simulink model "warp_timer"  (Simulink 7.1)
settings: Solver=ode45  StartTime=0.0  StopTime=1000  RelTol=1e-3
undefined symbols (not defined in the file): gcbh, xlBlockLoadCallback, xlGetSimulinkPeriod
libraries: xbsIndex_r4 x450
(part 4 of 5)

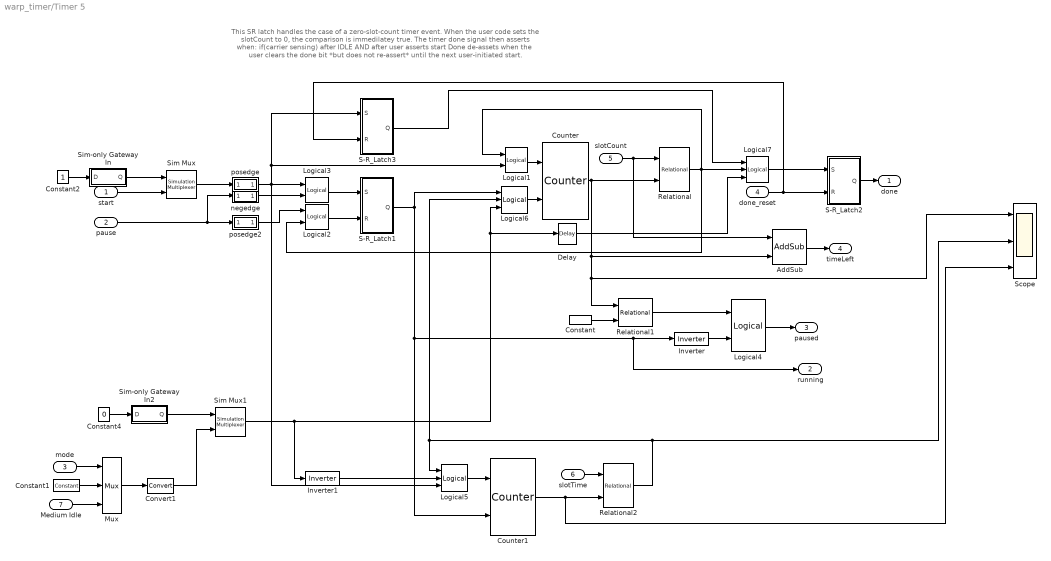
== system warp_timer/Timer 5 ==
  note: This SR latch handles the case of a zero-slot-count
      | timer event. When the user code sets the slotCount to 0,
      | the comparison is immedilatey true. The timer done
      | signal then asserts when:
      | if(carrier sensing) after IDLE AND
      | after user asserts start
      | Done de-assets when the user clears the done bit
      | *but does not re-assert* until the next user-initiated start.
  start : Inport  OutDataType=sfix(16)  OutScaling=2^0
  pause : Inport  Port=2  OutDataType=sfix(16)  OutScaling=2^0
  mode : Inport  Port=3  OutDataType=sfix(16)  OutScaling=2^0
  done_reset : Inport  Port=4  OutDataType=sfix(16)  OutScaling=2^0
  slotCount : Inport  Port=5  OutDataType=sfix(16)  OutScaling=2^0
  slotTime : Inport  Port=6  OutDataType=sfix(16)  OutScaling=2^0
  Medium Idle : Inport  Port=7  OutDataType=sfix(16)  OutScaling=2^0
  AddSub : xbsIndex_r4/AddSub  mode=Subtraction  use_carryin=off  use_carryout=off  en=off  latency=0  precision=User Defined  arith_type=Unsigned  n_bits=32  bin_pt=0  quantization=Truncate  overflow=Wrap  dbl_ovrd=off  use_behavioral_HDL=off  pipelined=off  use_rpm=on  hw_selection=Fabric  block_type=addsub
      settings: xl_area=[16 0 0 32 0 0 0]  block_version=8.2
  Constant : xbsIndex_r4/Constant  arith_type=Unsigned  const=0  n_bits=32  bin_pt=0  explicit_period=off  period=1  equ=P=C  opselect=C  inp2=PCIN>>17  opr=+  inp1=P  carry=CIN  dbl_ovrd=off  block_type=constant
      settings: block_version=10.1.2
  Constant1 : xbsIndex_r4/Constant  arith_type=Unsigned  const=1  n_bits=1  bin_pt=0  explicit_period=off  period=1  equ=P=C  opselect=C  inp2=PCIN>>17  opr=+  inp1=P  carry=CIN  dbl_ovrd=off  block_type=constant
      settings: block_version=8.2
  Constant2 : Constant  OutDataType=sfix(16)  OutScaling=2^0
  Constant4 : Constant  Value=0  OutDataType=sfix(16)  OutScaling=2^0
  Convert1 : xbsIndex_r4/Convert  arith_type=Boolean  n_bits=16  bin_pt=14  quantization=Truncate  overflow=Wrap  latency=0  dbl_ovrd=off  pipeline=off  block_type=convert
      settings: xl_area=[0 0 0 0 0 0 0]  block_version=8.2
  Counter : xbsIndex_r4/Counter  cnt_type=Free Running  cnt_to=Inf  operation=Up  start_count=0  cnt_by_val=1  arith_type=Unsigned  n_bits=32  bin_pt=0  load_pin=off  rst=on  en=on  explicit_period=on  period=1  dbl_ovrd=off  use_behavioral_HDL=off  use_rpm=off  implementation=Fabric  block_type=counter
      settings: xl_area=[17 32 0 32 0 0 0]  block_version=8.2
  Counter1 : xbsIndex_r4/Counter  cnt_type=Free Running  cnt_to=Inf  operation=Up  start_count=0  cnt_by_val=1  arith_type=Unsigned  n_bits=16  bin_pt=0  load_pin=off  rst=on  en=on  explicit_period=on  period=1  dbl_ovrd=off  use_behavioral_HDL=off  use_rpm=off  implementation=Fabric  block_type=counter
      settings: xl_area=[17 32 0 32 0 0 0]  block_version=8.2
  Delay : xbsIndex_r4/Delay  en=off  latency=1  dbl_ovrd=off  reg_retiming=off  block_type=delay
  Inverter : xbsIndex_r4/Inverter  en=off  latency=0  dbl_ovrd=off  block_type=inv
      settings: xl_area=[0 0 0 0 0 0 0]  block_version=10.1.2
  Inverter1 : xbsIndex_r4/Inverter  en=off  latency=0  dbl_ovrd=off  block_type=inv
      settings: xl_area=[0 0 0 0 0 0 0]  block_version=10.1.2
  Logical1 : xbsIndex_r4/Logical  logical_function=OR  inputs=2  en=off  latency=0  precision=Full  arith_type=Unsigned  n_bits=16  bin_pt=0  align_bp=on  dbl_ovrd=off  block_type=logical
      settings: xl_area=[1 0 0 1 0 0 0]  block_version=9.1.01
  Logical2 : xbsIndex_r4/Logical  logical_function=OR  inputs=2  en=off  latency=0  precision=Full  arith_type=Unsigned  n_bits=16  bin_pt=0  align_bp=on  dbl_ovrd=off  block_type=logical
      settings: xl_area=[1 0 0 1 0 0 0]  block_version=9.1.01
  Logical3 : xbsIndex_r4/Logical  logical_function=OR  inputs=2  en=off  latency=0  precision=Full  arith_type=Unsigned  n_bits=16  bin_pt=0  align_bp=on  dbl_ovrd=off  block_type=logical
      settings: xl_area=[1 0 0 1 0 0 0]  block_version=9.1.01
  Logical4 : xbsIndex_r4/Logical  logical_function=AND  inputs=2  en=off  latency=0  precision=Full  arith_type=Unsigned  n_bits=16  bin_pt=0  align_bp=on  dbl_ovrd=off  block_type=logical
      settings: xl_area=[1 0 0 1 0 0 0]  block_version=10.1.2
  Logical5 : xbsIndex_r4/Logical  logical_function=OR  inputs=3  en=off  latency=0  precision=Full  arith_type=Unsigned  n_bits=16  bin_pt=0  align_bp=on  dbl_ovrd=off  block_type=logical
      settings: xl_area=[1 0 0 1 0 0 0]  block_version=8.2
  Logical6 : xbsIndex_r4/Logical  logical_function=AND  inputs=3  en=off  latency=0  precision=Full  arith_type=Unsigned  n_bits=16  bin_pt=0  align_bp=on  dbl_ovrd=off  block_type=logical
      settings: xl_area=[1 0 0 1 0 0 0]  block_version=8.2
  Logical7 : xbsIndex_r4/Logical  logical_function=AND  inputs=3  en=off  latency=0  precision=Full  arith_type=Unsigned  n_bits=16  bin_pt=0  align_bp=on  dbl_ovrd=off  block_type=logical
      settings: xl_area=[1 0 0 1 0 0 0]  block_version=9.1.01
  Mux : xbsIndex_r4/Mux  inputs=2  en=off  latency=0  precision=Full  arith_type=Unsigned  n_bits=16  bin_pt=14  quantization=Truncate  overflow=Wrap  dbl_ovrd=off  block_type=mux
      settings: xl_area=[1 0 0 1 0 0 0]  block_version=8.2
  Relational : xbsIndex_r4/Relational  mode=a<=b  en=off  latency=0  dbl_ovrd=off  block_type=relational
      settings: xl_area=[8 0 0 16 0 0 0]  block_version=8.2
  Relational1 : xbsIndex_r4/Relational  mode=a>b  en=off  latency=0  dbl_ovrd=off  block_type=relational
      settings: xl_area=[16 1 0 32 0 0 0]  block_version=10.1.2
  Relational2 : xbsIndex_r4/Relational  mode=a<=b  en=off  latency=0  dbl_ovrd=off  block_type=relational
      settings: xl_area=[8 0 0 16 0 0 0]  block_version=8.2
  S-R_Latch1 : Subsystem
  S-R_Latch2 : Subsystem
  S-R_Latch3 : Subsystem
  Scope : Scope  NumInputPorts=3
      settings: YMin=-5~-5~-5  YMax=5~5~5
  Sim Mux : xbsIndex_r4/Simulation Multiplexer  sim_sel=1  hw_sel=2  block_type=simmux
      settings: infoedit="Distinguish input subsystems as \"simulation only\" and \"generation only\".  The input specified For Simulation will be used during Simulink simulation.  The input specified For Generation will be used during code generation.  This block will typically be used on the output of a HW Co-Simulation, Black Box, or ModelSim subsystem.<P><P>Hardware Notes: This block costs nothing."  block_version=10.1.3
  Sim Mux1 : xbsIndex_r4/Simulation Multiplexer  sim_sel=1  hw_sel=2  block_type=simmux
      settings: infoedit="Distinguish input subsystems as \"simulation only\" and \"generation only\".  The input specified For Simulation will be used during Simulink simulation.  The input specified For Generation will be used during code generation.  This block will typically be used on the output of a HW Co-Simulation, Black Box, or ModelSim subsystem.<P><P>Hardware Notes: This block costs nothing."  block_version=10.1.3
  Sim-only Gateway In : Subsystem
  Sim-only Gateway In2 : Subsystem
  negedge : Subsystem
  posedge : Subsystem
  posedge2 : Subsystem
  done : Outport  OutDataType=sfix(16)  OutScaling=2^0
  running : Outport  Port=2  OutDataType=sfix(16)  OutScaling=2^0
  paused : Outport  Port=3  OutDataType=sfix(16)  OutScaling=2^0
  timeLeft : Outport  Port=4  OutDataType=sfix(16)  OutScaling=2^0
  wires:
  Delay/1 -> Logical7/3
  S-R_Latch3/1(Q) -> Logical7/1
  Logical7/1 -> S-R_Latch2/1(S)
  Sim-only Gateway In2/1(Q) -> Sim Mux1/1
  Constant4/1 -> Sim-only Gateway In2/1(D)
  Logical2/1 -> S-R_Latch1/2(R)
  posedge2/1(Out) -> Logical2/1
  Constant2/1 -> Sim-only Gateway In/1(D)
  Sim Mux1/1 -> Delay/1, Logical6/3, Inverter1/1
  Convert1/1 -> Sim Mux1/2
  Logical6/1 -> Counter/2
  Inverter1/1 -> Logical5/2
  Relational2/1 -> Scope/2, Logical6/2, Logical5/1
  Logical5/1 -> Counter1/1
  Counter1/1 -> Scope/3, Relational2/2
  slotTime/1 -> Relational2/1
  Sim-only Gateway In/1(Q) -> Sim Mux/1
  pause/1 -> negedge/1(In), posedge2/1(In)
  negedge/1(Out) -> Logical3/2
  Logical3/1 -> S-R_Latch1/1(S)
  posedge/1(Out) -> S-R_Latch3/1(S), Logical1/2, Logical5/3, Logical3/1
  done_reset/1 -> S-R_Latch3/2(R), S-R_Latch2/2(R)
  Relational/1 -> Logical7/2, Logical1/1, Logical2/2
  S-R_Latch2/1(Q) -> done/1
  Logical1/1 -> Counter/1
  Counter/1 -> Scope/1, Relational1/1, AddSub/2, Relational/2
  slotCount/1 -> Relational/1, AddSub/1
  S-R_Latch1/1(Q) -> Logical6/1, running/1, Inverter/1, Counter1/2
  Inverter/1 -> Logical4/2
  Relational1/1 -> Logical4/1
  Constant/1 -> Relational1/2
  AddSub/1 -> timeLeft/1
  Sim Mux/1 -> posedge/1(In)
  start/1 -> Sim Mux/2
  Logical4/1 -> paused/1
  Mux/1 -> Convert1/1
  Medium Idle/1 -> Mux/3
  Constant1/1 -> Mux/2
  mode/1 -> Mux/1

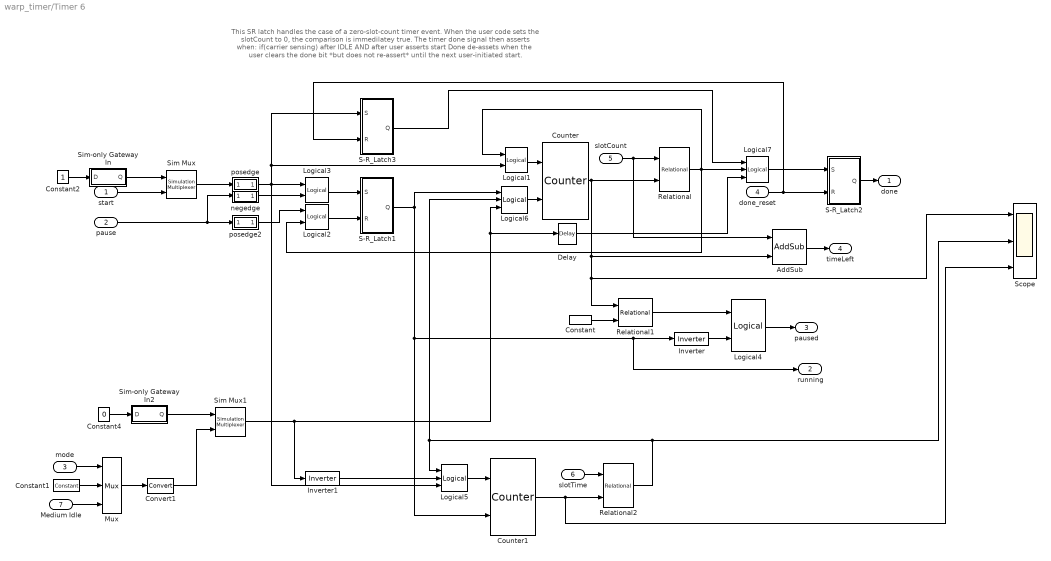
== system warp_timer/Timer 6 ==
  note: This SR latch handles the case of a zero-slot-count
      | timer event. When the user code sets the slotCount to 0,
      | the comparison is immedilatey true. The timer done
      | signal then asserts when:
      | if(carrier sensing) after IDLE AND
      | after user asserts start
      | Done de-assets when the user clears the done bit
      | *but does not re-assert* until the next user-initiated start.
  start : Inport  OutDataType=sfix(16)  OutScaling=2^0
  pause : Inport  Port=2  OutDataType=sfix(16)  OutScaling=2^0
  mode : Inport  Port=3  OutDataType=sfix(16)  OutScaling=2^0
  done_reset : Inport  Port=4  OutDataType=sfix(16)  OutScaling=2^0
  slotCount : Inport  Port=5  OutDataType=sfix(16)  OutScaling=2^0
  slotTime : Inport  Port=6  OutDataType=sfix(16)  OutScaling=2^0
  Medium Idle : Inport  Port=7  OutDataType=sfix(16)  OutScaling=2^0
  AddSub : xbsIndex_r4/AddSub  mode=Subtraction  use_carryin=off  use_carryout=off  en=off  latency=0  precision=User Defined  arith_type=Unsigned  n_bits=32  bin_pt=0  quantization=Truncate  overflow=Wrap  dbl_ovrd=off  use_behavioral_HDL=off  pipelined=off  use_rpm=on  hw_selection=Fabric  block_type=addsub
      settings: xl_area=[16 0 0 32 0 0 0]  block_version=8.2
  Constant : xbsIndex_r4/Constant  arith_type=Unsigned  const=0  n_bits=32  bin_pt=0  explicit_period=off  period=1  equ=P=C  opselect=C  inp2=PCIN>>17  opr=+  inp1=P  carry=CIN  dbl_ovrd=off  block_type=constant
      settings: block_version=10.1.2
  Constant1 : xbsIndex_r4/Constant  arith_type=Unsigned  const=1  n_bits=1  bin_pt=0  explicit_period=off  period=1  equ=P=C  opselect=C  inp2=PCIN>>17  opr=+  inp1=P  carry=CIN  dbl_ovrd=off  block_type=constant
      settings: block_version=8.2
  Constant2 : Constant  OutDataType=sfix(16)  OutScaling=2^0
  Constant4 : Constant  Value=0  OutDataType=sfix(16)  OutScaling=2^0
  Convert1 : xbsIndex_r4/Convert  arith_type=Boolean  n_bits=16  bin_pt=14  quantization=Truncate  overflow=Wrap  latency=0  dbl_ovrd=off  pipeline=off  block_type=convert
      settings: xl_area=[0 0 0 0 0 0 0]  block_version=8.2
  Counter : xbsIndex_r4/Counter  cnt_type=Free Running  cnt_to=Inf  operation=Up  start_count=0  cnt_by_val=1  arith_type=Unsigned  n_bits=32  bin_pt=0  load_pin=off  rst=on  en=on  explicit_period=on  period=1  dbl_ovrd=off  use_behavioral_HDL=off  use_rpm=off  implementation=Fabric  block_type=counter
      settings: xl_area=[17 32 0 32 0 0 0]  block_version=8.2
  Counter1 : xbsIndex_r4/Counter  cnt_type=Free Running  cnt_to=Inf  operation=Up  start_count=0  cnt_by_val=1  arith_type=Unsigned  n_bits=16  bin_pt=0  load_pin=off  rst=on  en=on  explicit_period=on  period=1  dbl_ovrd=off  use_behavioral_HDL=off  use_rpm=off  implementation=Fabric  block_type=counter
      settings: xl_area=[17 32 0 32 0 0 0]  block_version=8.2
  Delay : xbsIndex_r4/Delay  en=off  latency=1  dbl_ovrd=off  reg_retiming=off  block_type=delay
  Inverter : xbsIndex_r4/Inverter  en=off  latency=0  dbl_ovrd=off  block_type=inv
      settings: xl_area=[0 0 0 0 0 0 0]  block_version=10.1.2
  Inverter1 : xbsIndex_r4/Inverter  en=off  latency=0  dbl_ovrd=off  block_type=inv
      settings: xl_area=[0 0 0 0 0 0 0]  block_version=10.1.2
  Logical1 : xbsIndex_r4/Logical  logical_function=OR  inputs=2  en=off  latency=0  precision=Full  arith_type=Unsigned  n_bits=16  bin_pt=0  align_bp=on  dbl_ovrd=off  block_type=logical
      settings: xl_area=[1 0 0 1 0 0 0]  block_version=9.1.01
  Logical2 : xbsIndex_r4/Logical  logical_function=OR  inputs=2  en=off  latency=0  precision=Full  arith_type=Unsigned  n_bits=16  bin_pt=0  align_bp=on  dbl_ovrd=off  block_type=logical
      settings: xl_area=[1 0 0 1 0 0 0]  block_version=9.1.01
  Logical3 : xbsIndex_r4/Logical  logical_function=OR  inputs=2  en=off  latency=0  precision=Full  arith_type=Unsigned  n_bits=16  bin_pt=0  align_bp=on  dbl_ovrd=off  block_type=logical
      settings: xl_area=[1 0 0 1 0 0 0]  block_version=9.1.01
  Logical4 : xbsIndex_r4/Logical  logical_function=AND  inputs=2  en=off  latency=0  precision=Full  arith_type=Unsigned  n_bits=16  bin_pt=0  align_bp=on  dbl_ovrd=off  block_type=logical
      settings: xl_area=[1 0 0 1 0 0 0]  block_version=10.1.2
  Logical5 : xbsIndex_r4/Logical  logical_function=OR  inputs=3  en=off  latency=0  precision=Full  arith_type=Unsigned  n_bits=16  bin_pt=0  align_bp=on  dbl_ovrd=off  block_type=logical
      settings: xl_area=[1 0 0 1 0 0 0]  block_version=8.2
  Logical6 : xbsIndex_r4/Logical  logical_function=AND  inputs=3  en=off  latency=0  precision=Full  arith_type=Unsigned  n_bits=16  bin_pt=0  align_bp=on  dbl_ovrd=off  block_type=logical
      settings: xl_area=[1 0 0 1 0 0 0]  block_version=8.2
  Logical7 : xbsIndex_r4/Logical  logical_function=AND  inputs=3  en=off  latency=0  precision=Full  arith_type=Unsigned  n_bits=16  bin_pt=0  align_bp=on  dbl_ovrd=off  block_type=logical
      settings: xl_area=[1 0 0 1 0 0 0]  block_version=9.1.01
  Mux : xbsIndex_r4/Mux  inputs=2  en=off  latency=0  precision=Full  arith_type=Unsigned  n_bits=16  bin_pt=14  quantization=Truncate  overflow=Wrap  dbl_ovrd=off  block_type=mux
      settings: xl_area=[1 0 0 1 0 0 0]  block_version=8.2
  Relational : xbsIndex_r4/Relational  mode=a<=b  en=off  latency=0  dbl_ovrd=off  block_type=relational
      settings: xl_area=[8 0 0 16 0 0 0]  block_version=8.2
  Relational1 : xbsIndex_r4/Relational  mode=a>b  en=off  latency=0  dbl_ovrd=off  block_type=relational
      settings: xl_area=[16 1 0 32 0 0 0]  block_version=10.1.2
  Relational2 : xbsIndex_r4/Relational  mode=a<=b  en=off  latency=0  dbl_ovrd=off  block_type=relational
      settings: xl_area=[8 0 0 16 0 0 0]  block_version=8.2
  S-R_Latch1 : Subsystem
  S-R_Latch2 : Subsystem
  S-R_Latch3 : Subsystem
  Scope : Scope  NumInputPorts=3
      settings: YMin=-5~-5~-5  YMax=5~5~5
  Sim Mux : xbsIndex_r4/Simulation Multiplexer  sim_sel=1  hw_sel=2  block_type=simmux
      settings: infoedit="Distinguish input subsystems as \"simulation only\" and \"generation only\".  The input specified For Simulation will be used during Simulink simulation.  The input specified For Generation will be used during code generation.  This block will typically be used on the output of a HW Co-Simulation, Black Box, or ModelSim subsystem.<P><P>Hardware Notes: This block costs nothing."  block_version=10.1.3
  Sim Mux1 : xbsIndex_r4/Simulation Multiplexer  sim_sel=1  hw_sel=2  block_type=simmux
      settings: infoedit="Distinguish input subsystems as \"simulation only\" and \"generation only\".  The input specified For Simulation will be used during Simulink simulation.  The input specified For Generation will be used during code generation.  This block will typically be used on the output of a HW Co-Simulation, Black Box, or ModelSim subsystem.<P><P>Hardware Notes: This block costs nothing."  block_version=10.1.3
  Sim-only Gateway In : Subsystem
  Sim-only Gateway In2 : Subsystem
  negedge : Subsystem
  posedge : Subsystem
  posedge2 : Subsystem
  done : Outport  OutDataType=sfix(16)  OutScaling=2^0
  running : Outport  Port=2  OutDataType=sfix(16)  OutScaling=2^0
  paused : Outport  Port=3  OutDataType=sfix(16)  OutScaling=2^0
  timeLeft : Outport  Port=4  OutDataType=sfix(16)  OutScaling=2^0
  wires:
  mode/1 -> Mux/1
  Constant1/1 -> Mux/2
  Medium Idle/1 -> Mux/3
  Mux/1 -> Convert1/1
  Logical4/1 -> paused/1
  start/1 -> Sim Mux/2
  Sim Mux/1 -> posedge/1(In)
  AddSub/1 -> timeLeft/1
  Constant/1 -> Relational1/2
  Relational1/1 -> Logical4/1
  Inverter/1 -> Logical4/2
  S-R_Latch1/1(Q) -> Counter1/2, Inverter/1, running/1, Logical6/1
  slotCount/1 -> AddSub/1, Relational/1
  Counter/1 -> Relational/2, AddSub/2, Relational1/1, Scope/1
  Logical1/1 -> Counter/1
  S-R_Latch2/1(Q) -> done/1
  Relational/1 -> Logical2/2, Logical1/1, Logical7/2
  done_reset/1 -> S-R_Latch2/2(R), S-R_Latch3/2(R)
  posedge/1(Out) -> Logical3/1, Logical5/3, Logical1/2, S-R_Latch3/1(S)
  Logical3/1 -> S-R_Latch1/1(S)
  negedge/1(Out) -> Logical3/2
  pause/1 -> posedge2/1(In), negedge/1(In)
  Sim-only Gateway In/1(Q) -> Sim Mux/1
  slotTime/1 -> Relational2/1
  Counter1/1 -> Relational2/2, Scope/3
  Logical5/1 -> Counter1/1
  Relational2/1 -> Logical5/1, Logical6/2, Scope/2
  Inverter1/1 -> Logical5/2
  Logical6/1 -> Counter/2
  Convert1/1 -> Sim Mux1/2
  Sim Mux1/1 -> Inverter1/1, Logical6/3, Delay/1
  Constant2/1 -> Sim-only Gateway In/1(D)
  posedge2/1(Out) -> Logical2/1
  Logical2/1 -> S-R_Latch1/2(R)
  Constant4/1 -> Sim-only Gateway In2/1(D)
  Sim-only Gateway In2/1(Q) -> Sim Mux1/1
  Logical7/1 -> S-R_Latch2/1(S)
  S-R_Latch3/1(Q) -> Logical7/1
  Delay/1 -> Logical7/3

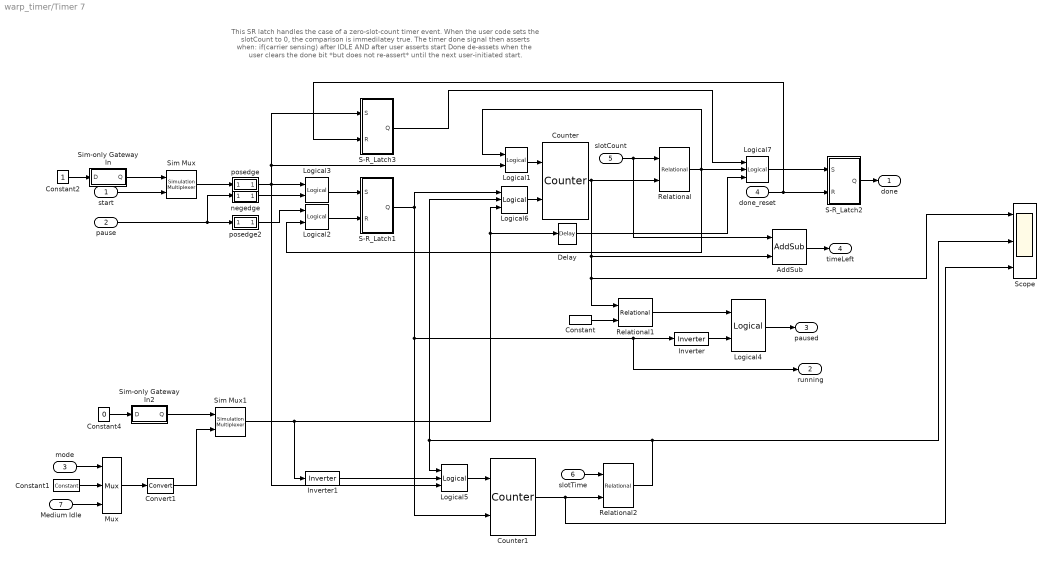
== system warp_timer/Timer 7 ==
  note: This SR latch handles the case of a zero-slot-count
      | timer event. When the user code sets the slotCount to 0,
      | the comparison is immedilatey true. The timer done
      | signal then asserts when:
      | if(carrier sensing) after IDLE AND
      | after user asserts start
      | Done de-assets when the user clears the done bit
      | *but does not re-assert* until the next user-initiated start.
  start : Inport  OutDataType=sfix(16)  OutScaling=2^0
  pause : Inport  Port=2  OutDataType=sfix(16)  OutScaling=2^0
  mode : Inport  Port=3  OutDataType=sfix(16)  OutScaling=2^0
  done_reset : Inport  Port=4  OutDataType=sfix(16)  OutScaling=2^0
  slotCount : Inport  Port=5  OutDataType=sfix(16)  OutScaling=2^0
  slotTime : Inport  Port=6  OutDataType=sfix(16)  OutScaling=2^0
  Medium Idle : Inport  Port=7  OutDataType=sfix(16)  OutScaling=2^0
  AddSub : xbsIndex_r4/AddSub  mode=Subtraction  use_carryin=off  use_carryout=off  en=off  latency=0  precision=User Defined  arith_type=Unsigned  n_bits=32  bin_pt=0  quantization=Truncate  overflow=Wrap  dbl_ovrd=off  use_behavioral_HDL=off  pipelined=off  use_rpm=on  hw_selection=Fabric  block_type=addsub
      settings: xl_area=[16 0 0 32 0 0 0]  block_version=8.2
  Constant : xbsIndex_r4/Constant  arith_type=Unsigned  const=0  n_bits=32  bin_pt=0  explicit_period=off  period=1  equ=P=C  opselect=C  inp2=PCIN>>17  opr=+  inp1=P  carry=CIN  dbl_ovrd=off  block_type=constant
      settings: block_version=10.1.2
  Constant1 : xbsIndex_r4/Constant  arith_type=Unsigned  const=1  n_bits=1  bin_pt=0  explicit_period=off  period=1  equ=P=C  opselect=C  inp2=PCIN>>17  opr=+  inp1=P  carry=CIN  dbl_ovrd=off  block_type=constant
      settings: block_version=8.2
  Constant2 : Constant  OutDataType=sfix(16)  OutScaling=2^0
  Constant4 : Constant  Value=0  OutDataType=sfix(16)  OutScaling=2^0
  Convert1 : xbsIndex_r4/Convert  arith_type=Boolean  n_bits=16  bin_pt=14  quantization=Truncate  overflow=Wrap  latency=0  dbl_ovrd=off  pipeline=off  block_type=convert
      settings: xl_area=[0 0 0 0 0 0 0]  block_version=8.2
  Counter : xbsIndex_r4/Counter  cnt_type=Free Running  cnt_to=Inf  operation=Up  start_count=0  cnt_by_val=1  arith_type=Unsigned  n_bits=32  bin_pt=0  load_pin=off  rst=on  en=on  explicit_period=on  period=1  dbl_ovrd=off  use_behavioral_HDL=off  use_rpm=off  implementation=Fabric  block_type=counter
      settings: xl_area=[17 32 0 32 0 0 0]  block_version=8.2
  Counter1 : xbsIndex_r4/Counter  cnt_type=Free Running  cnt_to=Inf  operation=Up  start_count=0  cnt_by_val=1  arith_type=Unsigned  n_bits=16  bin_pt=0  load_pin=off  rst=on  en=on  explicit_period=on  period=1  dbl_ovrd=off  use_behavioral_HDL=off  use_rpm=off  implementation=Fabric  block_type=counter
      settings: xl_area=[17 32 0 32 0 0 0]  block_version=8.2
  Delay : xbsIndex_r4/Delay  en=off  latency=1  dbl_ovrd=off  reg_retiming=off  block_type=delay
  Inverter : xbsIndex_r4/Inverter  en=off  latency=0  dbl_ovrd=off  block_type=inv
      settings: xl_area=[0 0 0 0 0 0 0]  block_version=10.1.2
  Inverter1 : xbsIndex_r4/Inverter  en=off  latency=0  dbl_ovrd=off  block_type=inv
      settings: xl_area=[0 0 0 0 0 0 0]  block_version=10.1.2
  Logical1 : xbsIndex_r4/Logical  logical_function=OR  inputs=2  en=off  latency=0  precision=Full  arith_type=Unsigned  n_bits=16  bin_pt=0  align_bp=on  dbl_ovrd=off  block_type=logical
      settings: xl_area=[1 0 0 1 0 0 0]  block_version=9.1.01
  Logical2 : xbsIndex_r4/Logical  logical_function=OR  inputs=2  en=off  latency=0  precision=Full  arith_type=Unsigned  n_bits=16  bin_pt=0  align_bp=on  dbl_ovrd=off  block_type=logical
      settings: xl_area=[1 0 0 1 0 0 0]  block_version=9.1.01
  Logical3 : xbsIndex_r4/Logical  logical_function=OR  inputs=2  en=off  latency=0  precision=Full  arith_type=Unsigned  n_bits=16  bin_pt=0  align_bp=on  dbl_ovrd=off  block_type=logical
      settings: xl_area=[1 0 0 1 0 0 0]  block_version=9.1.01
  Logical4 : xbsIndex_r4/Logical  logical_function=AND  inputs=2  en=off  latency=0  precision=Full  arith_type=Unsigned  n_bits=16  bin_pt=0  align_bp=on  dbl_ovrd=off  block_type=logical
      settings: xl_area=[1 0 0 1 0 0 0]  block_version=10.1.2
  Logical5 : xbsIndex_r4/Logical  logical_function=OR  inputs=3  en=off  latency=0  precision=Full  arith_type=Unsigned  n_bits=16  bin_pt=0  align_bp=on  dbl_ovrd=off  block_type=logical
      settings: xl_area=[1 0 0 1 0 0 0]  block_version=8.2
  Logical6 : xbsIndex_r4/Logical  logical_function=AND  inputs=3  en=off  latency=0  precision=Full  arith_type=Unsigned  n_bits=16  bin_pt=0  align_bp=on  dbl_ovrd=off  block_type=logical
      settings: xl_area=[1 0 0 1 0 0 0]  block_version=8.2
  Logical7 : xbsIndex_r4/Logical  logical_function=AND  inputs=3  en=off  latency=0  precision=Full  arith_type=Unsigned  n_bits=16  bin_pt=0  align_bp=on  dbl_ovrd=off  block_type=logical
      settings: xl_area=[1 0 0 1 0 0 0]  block_version=9.1.01
  Mux : xbsIndex_r4/Mux  inputs=2  en=off  latency=0  precision=Full  arith_type=Unsigned  n_bits=16  bin_pt=14  quantization=Truncate  overflow=Wrap  dbl_ovrd=off  block_type=mux
      settings: xl_area=[1 0 0 1 0 0 0]  block_version=8.2
  Relational : xbsIndex_r4/Relational  mode=a<=b  en=off  latency=0  dbl_ovrd=off  block_type=relational
      settings: xl_area=[8 0 0 16 0 0 0]  block_version=8.2
  Relational1 : xbsIndex_r4/Relational  mode=a>b  en=off  latency=0  dbl_ovrd=off  block_type=relational
      settings: xl_area=[16 1 0 32 0 0 0]  block_version=10.1.2
  Relational2 : xbsIndex_r4/Relational  mode=a<=b  en=off  latency=0  dbl_ovrd=off  block_type=relational
      settings: xl_area=[8 0 0 16 0 0 0]  block_version=8.2
  S-R_Latch1 : Subsystem
  S-R_Latch2 : Subsystem
  S-R_Latch3 : Subsystem
  Scope : Scope  NumInputPorts=3
      settings: YMin=-5~-5~-5  YMax=5~5~5
  Sim Mux : xbsIndex_r4/Simulation Multiplexer  sim_sel=1  hw_sel=2  block_type=simmux
      settings: infoedit="Distinguish input subsystems as \"simulation only\" and \"generation only\".  The input specified For Simulation will be used during Simulink simulation.  The input specified For Generation will be used during code generation.  This block will typically be used on the output of a HW Co-Simulation, Black Box, or ModelSim subsystem.<P><P>Hardware Notes: This block costs nothing."  block_version=10.1.3
  Sim Mux1 : xbsIndex_r4/Simulation Multiplexer  sim_sel=1  hw_sel=2  block_type=simmux
      settings: infoedit="Distinguish input subsystems as \"simulation only\" and \"generation only\".  The input specified For Simulation will be used during Simulink simulation.  The input specified For Generation will be used during code generation.  This block will typically be used on the output of a HW Co-Simulation, Black Box, or ModelSim subsystem.<P><P>Hardware Notes: This block costs nothing."  block_version=10.1.3
  Sim-only Gateway In : Subsystem
  Sim-only Gateway In2 : Subsystem
  negedge : Subsystem
  posedge : Subsystem
  posedge2 : Subsystem
  done : Outport  OutDataType=sfix(16)  OutScaling=2^0
  running : Outport  Port=2  OutDataType=sfix(16)  OutScaling=2^0
  paused : Outport  Port=3  OutDataType=sfix(16)  OutScaling=2^0
  timeLeft : Outport  Port=4  OutDataType=sfix(16)  OutScaling=2^0
  wires:
  Delay/1 -> Logical7/3
  S-R_Latch3/1(Q) -> Logical7/1
  Logical7/1 -> S-R_Latch2/1(S)
  Sim-only Gateway In2/1(Q) -> Sim Mux1/1
  Constant4/1 -> Sim-only Gateway In2/1(D)
  Logical2/1 -> S-R_Latch1/2(R)
  posedge2/1(Out) -> Logical2/1
  Constant2/1 -> Sim-only Gateway In/1(D)
  Sim Mux1/1 -> Delay/1, Logical6/3, Inverter1/1
  Convert1/1 -> Sim Mux1/2
  Logical6/1 -> Counter/2
  Inverter1/1 -> Logical5/2
  Relational2/1 -> Scope/2, Logical6/2, Logical5/1
  Logical5/1 -> Counter1/1
  Counter1/1 -> Scope/3, Relational2/2
  slotTime/1 -> Relational2/1
  Sim-only Gateway In/1(Q) -> Sim Mux/1
  pause/1 -> negedge/1(In), posedge2/1(In)
  negedge/1(Out) -> Logical3/2
  Logical3/1 -> S-R_Latch1/1(S)
  posedge/1(Out) -> S-R_Latch3/1(S), Logical1/2, Logical5/3, Logical3/1
  done_reset/1 -> S-R_Latch3/2(R), S-R_Latch2/2(R)
  Relational/1 -> Logical7/2, Logical1/1, Logical2/2
  S-R_Latch2/1(Q) -> done/1
  Logical1/1 -> Counter/1
  Counter/1 -> Scope/1, Relational1/1, AddSub/2, Relational/2
  slotCount/1 -> Relational/1, AddSub/1
  S-R_Latch1/1(Q) -> Logical6/1, running/1, Inverter/1, Counter1/2
  Inverter/1 -> Logical4/2
  Relational1/1 -> Logical4/1
  Constant/1 -> Relational1/2
  AddSub/1 -> timeLeft/1
  Sim Mux/1 -> posedge/1(In)
  start/1 -> Sim Mux/2
  Logical4/1 -> paused/1
  Mux/1 -> Convert1/1
  Medium Idle/1 -> Mux/3
  Constant1/1 -> Mux/2
  mode/1 -> Mux/1

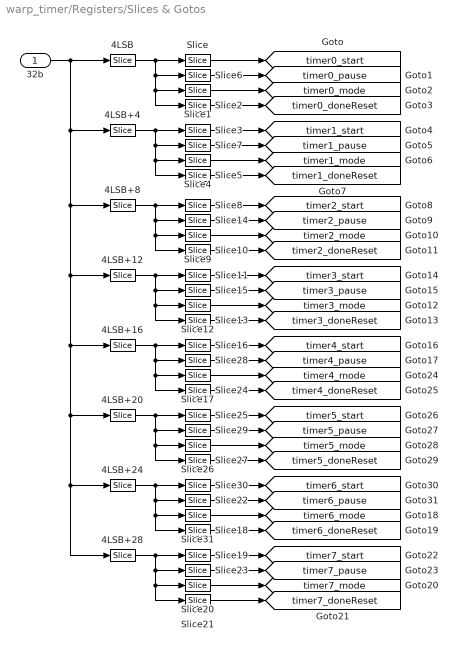
== system warp_timer/Registers/Slices & Gotos ==
  32b : Inport
  4LSB : xbsIndex_r4/Slice  nbits=4  boolean_output=off  mode=Lower Bit Location + Width  bit1=0  base1=LSB of Input  bit0=0  base0=LSB of Input  dbl_ovrd=off  block_type=slice
      settings: infoedit="Extracts a given range of bits from each input sample and presents it at the output.  The output type is ordinarily unsigned with binary point at zero, but can be Boolean when the slice is one bit wide.<P><P>Hardware notes: In hardware this block costs nothing."  block_version=9.1.01
  4LSB+12 : xbsIndex_r4/Slice  nbits=4  boolean_output=off  mode=Lower Bit Location + Width  bit1=0  base1=LSB of Input  bit0=12  base0=LSB of Input  dbl_ovrd=off  block_type=slice
      settings: infoedit="Extracts a given range of bits from each input sample and presents it at the output.  The output type is ordinarily unsigned with binary point at zero, but can be Boolean when the slice is one bit wide.<P><P>Hardware notes: In hardware this block costs nothing."  block_version=9.1.01
  4LSB+16 : xbsIndex_r4/Slice  nbits=4  boolean_output=off  mode=Lower Bit Location + Width  bit1=0  base1=LSB of Input  bit0=16  base0=LSB of Input  dbl_ovrd=off  block_type=slice
      settings: infoedit="Extracts a given range of bits from each input sample and presents it at the output.  The output type is ordinarily unsigned with binary point at zero, but can be Boolean when the slice is one bit wide.<P><P>Hardware notes: In hardware this block costs nothing."  block_version=9.1.01
  4LSB+20 : xbsIndex_r4/Slice  nbits=4  boolean_output=off  mode=Lower Bit Location + Width  bit1=0  base1=LSB of Input  bit0=20  base0=LSB of Input  dbl_ovrd=off  block_type=slice
      settings: infoedit="Extracts a given range of bits from each input sample and presents it at the output.  The output type is ordinarily unsigned with binary point at zero, but can be Boolean when the slice is one bit wide.<P><P>Hardware notes: In hardware this block costs nothing."  block_version=9.1.01
  4LSB+24 : xbsIndex_r4/Slice  nbits=4  boolean_output=off  mode=Lower Bit Location + Width  bit1=0  base1=LSB of Input  bit0=24  base0=LSB of Input  dbl_ovrd=off  block_type=slice
      settings: infoedit="Extracts a given range of bits from each input sample and presents it at the output.  The output type is ordinarily unsigned with binary point at zero, but can be Boolean when the slice is one bit wide.<P><P>Hardware notes: In hardware this block costs nothing."  block_version=9.1.01
  4LSB+28 : xbsIndex_r4/Slice  nbits=4  boolean_output=off  mode=Lower Bit Location + Width  bit1=0  base1=LSB of Input  bit0=28  base0=LSB of Input  dbl_ovrd=off  block_type=slice
      settings: infoedit="Extracts a given range of bits from each input sample and presents it at the output.  The output type is ordinarily unsigned with binary point at zero, but can be Boolean when the slice is one bit wide.<P><P>Hardware notes: In hardware this block costs nothing."  block_version=9.1.01
  4LSB+4 : xbsIndex_r4/Slice  nbits=4  boolean_output=off  mode=Lower Bit Location + Width  bit1=0  base1=LSB of Input  bit0=4  base0=LSB of Input  dbl_ovrd=off  block_type=slice
      settings: infoedit="Extracts a given range of bits from each input sample and presents it at the output.  The output type is ordinarily unsigned with binary point at zero, but can be Boolean when the slice is one bit wide.<P><P>Hardware notes: In hardware this block costs nothing."  block_version=9.1.01
  4LSB+8 : xbsIndex_r4/Slice  nbits=4  boolean_output=off  mode=Lower Bit Location + Width  bit1=0  base1=LSB of Input  bit0=8  base0=LSB of Input  dbl_ovrd=off  block_type=slice
      settings: infoedit="Extracts a given range of bits from each input sample and presents it at the output.  The output type is ordinarily unsigned with binary point at zero, but can be Boolean when the slice is one bit wide.<P><P>Hardware notes: In hardware this block costs nothing."  block_version=9.1.01
  Slice{,3,8,11,16,19,25,30} (8 alike) : xbsIndex_r4/Slice  nbits=1  boolean_output=on  mode=Lower Bit Location + Width  bit1=0  base1=LSB of Input  bit0=0  base0=LSB of Input  dbl_ovrd=off  block_type=slice
      settings: infoedit="Extracts a given range of bits from each input sample and presents it at the output.  The output type is ordinarily unsigned with binary point at zero, but can be Boolean when the slice is one bit wide.<P><P>Hardware notes: In hardware this block costs nothing."  block_version=9.1.01
  Slice{1,4,9,12,17,20,26,31} (8 alike) : xbsIndex_r4/Slice  nbits=1  boolean_output=on  mode=Lower Bit Location + Width  bit1=0  base1=LSB of Input  bit0=2  base0=LSB of Input  dbl_ovrd=off  block_type=slice
      settings: infoedit="Extracts a given range of bits from each input sample and presents it at the output.  The output type is ordinarily unsigned with binary point at zero, but can be Boolean when the slice is one bit wide.<P><P>Hardware notes: In hardware this block costs nothing."  block_version=9.1.01
  Slice{2,5,10,13,18,21,24,27} (8 alike) : xbsIndex_r4/Slice  nbits=1  boolean_output=on  mode=Lower Bit Location + Width  bit1=0  base1=LSB of Input  bit0=3  base0=LSB of Input  dbl_ovrd=off  block_type=slice
      settings: infoedit="Extracts a given range of bits from each input sample and presents it at the output.  The output type is ordinarily unsigned with binary point at zero, but can be Boolean when the slice is one bit wide.<P><P>Hardware notes: In hardware this block costs nothing."  block_version=9.1.01
  Slice{6..7,14..15,22..23,28..29} (8 alike) : xbsIndex_r4/Slice  nbits=1  boolean_output=on  mode=Lower Bit Location + Width  bit1=0  base1=LSB of Input  bit0=1  base0=LSB of Input  dbl_ovrd=off  block_type=slice
      settings: infoedit="Extracts a given range of bits from each input sample and presents it at the output.  The output type is ordinarily unsigned with binary point at zero, but can be Boolean when the slice is one bit wide.<P><P>Hardware notes: In hardware this block costs nothing."  block_version=9.1.01
  tag scope: timer0_doneReset=global, timer0_mode=global, timer0_pause=global, timer0_start=global, timer1_doneReset=global, timer1_mode=global, timer1_pause=global, timer1_start=global, timer2_doneReset=global, timer2_mode=global, timer2_pause=global, timer2_start=global, timer3_doneReset=global, timer3_mode=global, timer3_pause=global, timer3_start=global, timer4_doneReset=global, timer4_mode=global, timer4_pause=global, timer4_start=global, timer5_doneReset=global, timer5_mode=global, timer5_pause=global, timer5_start=global, timer6_doneReset=global, timer6_mode=global, timer6_pause=global, timer6_start=global, timer7_doneReset=global, timer7_mode=global, timer7_pause=global, timer7_start=global
  wires:
  32b/1 -> 4LSB+28/1, 4LSB+24/1, 4LSB+20/1, 4LSB+16/1, 4LSB+12/1, 4LSB+8/1, 4LSB+4/1, 4LSB/1
  4LSB/1 -> Slice/1, Slice6/1, Slice2/1, Slice1/1
  4LSB+4/1 -> Slice4/1, Slice5/1, Slice7/1, Slice3/1
  Slice/1 -> [timer0_start]
  Slice6/1 -> [timer0_pause]
  Slice1/1 -> [timer0_mode]
  Slice2/1 -> [timer0_doneReset]
  Slice3/1 -> [timer1_start]
  Slice7/1 -> [timer1_pause]
  Slice4/1 -> [timer1_mode]
  Slice5/1 -> [timer1_doneReset]
  4LSB+8/1 -> Slice9/1, Slice10/1, Slice14/1, Slice8/1
  4LSB+12/1 -> Slice11/1, Slice15/1, Slice13/1, Slice12/1
  Slice8/1 -> [timer2_start]
  Slice14/1 -> [timer2_pause]
  Slice9/1 -> [timer2_mode]
  Slice10/1 -> [timer2_doneReset]
  Slice11/1 -> [timer3_start]
  Slice15/1 -> [timer3_pause]
  Slice12/1 -> [timer3_mode]
  Slice13/1 -> [timer3_doneReset]
  4LSB+16/1 -> Slice17/1, Slice24/1, Slice28/1, Slice16/1
  4LSB+20/1 -> Slice25/1, Slice29/1, Slice27/1, Slice26/1
  Slice16/1 -> [timer4_start]
  Slice28/1 -> [timer4_pause]
  Slice17/1 -> [timer4_mode]
  Slice24/1 -> [timer4_doneReset]
  Slice25/1 -> [timer5_start]
  Slice29/1 -> [timer5_pause]
  Slice26/1 -> [timer5_mode]
  Slice27/1 -> [timer5_doneReset]
  4LSB+24/1 -> Slice30/1, Slice22/1, Slice18/1, Slice31/1
  4LSB+28/1 -> Slice20/1, Slice21/1, Slice23/1, Slice19/1
  Slice30/1 -> [timer6_start]
  Slice22/1 -> [timer6_pause]
  Slice31/1 -> [timer6_mode]
  Slice18/1 -> [timer6_doneReset]
  Slice19/1 -> [timer7_start]
  Slice23/1 -> [timer7_pause]
  Slice20/1 -> [timer7_mode]
  Slice21/1 -> [timer7_doneReset]

== system warp_timer/Timer 0/S-R_Latch1 ==
  S : Inport  OutDataType=sfix(16)  OutScaling=2^0
  R : Inport  Port=2  OutDataType=sfix(16)  OutScaling=2^0
  Inverter : xbsIndex_r4/Inverter  en=off  latency=0  dbl_ovrd=off  block_type=inv
      settings: xl_area=[0 0 0 0 0 0 0]  block_version=VER_STRING_GOES_HERE
  Register : xbsIndex_r4/Register  init=0  rst=on  en=on  dbl_ovrd=off  block_type=register
      settings: xl_area=[1 1 0 0 0 0 0]  block_version=VER_STRING_GOES_HERE
  Q : Outport  OutDataType=sfix(16)  OutScaling=2^0
  wires:
  R/1 -> Register/2
  S/1 -> Register/1
  Inverter/1 -> Register/3
  Register/1 -> Q/1, Inverter/1

== system warp_timer/Timer 0/S-R_Latch2 ==
  S : Inport  OutDataType=sfix(16)  OutScaling=2^0
  R : Inport  Port=2  OutDataType=sfix(16)  OutScaling=2^0
  Inverter : xbsIndex_r4/Inverter  en=off  latency=0  dbl_ovrd=off  block_type=inv
      settings: xl_area=[0 0 0 0 0 0 0]  block_version=VER_STRING_GOES_HERE
  Register : xbsIndex_r4/Register  init=0  rst=on  en=on  dbl_ovrd=off  block_type=register
      settings: xl_area=[1 1 0 0 0 0 0]  block_version=VER_STRING_GOES_HERE
  Q : Outport  OutDataType=sfix(16)  OutScaling=2^0
  wires:
  Register/1 -> Inverter/1, Q/1
  Inverter/1 -> Register/3
  S/1 -> Register/1
  R/1 -> Register/2

== system warp_timer/Timer 0/S-R_Latch3 ==
  S : Inport  OutDataType=sfix(16)  OutScaling=2^0
  R : Inport  Port=2  OutDataType=sfix(16)  OutScaling=2^0
  Inverter : xbsIndex_r4/Inverter  en=off  latency=0  dbl_ovrd=off  block_type=inv
      settings: xl_area=[0 0 0 0 0 0 0]  block_version=VER_STRING_GOES_HERE
  Register : xbsIndex_r4/Register  init=0  rst=on  en=on  dbl_ovrd=off  block_type=register
      settings: xl_area=[1 1 0 0 0 0 0]  block_version=VER_STRING_GOES_HERE
  Q : Outport  OutDataType=sfix(16)  OutScaling=2^0
  wires:
  Register/1 -> Inverter/1, Q/1
  Inverter/1 -> Register/3
  S/1 -> Register/1
  R/1 -> Register/2

== system warp_timer/Timer 0/Sim-only Gateway In ==
  D : Inport  OutDataType=sfix(16)  OutScaling=2^0
  Disregard Subsystem : xbsIndex_r4/Disregard Subsystem  Tag=discardX  block_type=disregard
      settings: block_version=10.1.3
  Gateway In : xbsIndex_r4/Gateway In  arith_type=Boolean  n_bits=1  bin_pt=0  quantization="Round  (unbiased: +/- Inf)"  overflow=Saturate  period=1  dbl_ovrd=off  timing_constraint=None  locs_specified=off  LOCs={}  block_type=gatewayin
      settings: infoedit="Gateway in block.  Converts inputs of type Simulink integer, double and fixed point to  Xilinx fixed point type.<P><P>Hardware notes:  In hardware these blocks become top level input ports."  xl_area=[0 0 0 0 1 0 0]  block_version=10.1.3
  Q : Outport
  wires:
  D/1 -> Gateway In/1
  Gateway In/1 -> Q/1

== system warp_timer/Timer 0/Sim-only Gateway In2 ==
  D : Inport  OutDataType=sfix(16)  OutScaling=2^0
  Disregard Subsystem : xbsIndex_r4/Disregard Subsystem  Tag=discardX  block_type=disregard
      settings: block_version=10.1.3
  Gateway In : xbsIndex_r4/Gateway In  arith_type=Boolean  n_bits=1  bin_pt=0  quantization="Round  (unbiased: +/- Inf)"  overflow=Saturate  period=1  dbl_ovrd=off  timing_constraint=None  locs_specified=off  LOCs={}  block_type=gatewayin
      settings: infoedit="Gateway in block.  Converts inputs of type Simulink integer, double and fixed point to  Xilinx fixed point type.<P><P>Hardware notes:  In hardware these blocks become top level input ports."  xl_area=[0 0 0 0 1 0 0]  block_version=10.1.3
  Q : Outport
  wires:
  Gateway In/1 -> Q/1
  D/1 -> Gateway In/1

== system warp_timer/Timer 0/negedge ==
  In : Inport  OutDataType=sfix(16)  OutScaling=2^0
  Delay : xbsIndex_r4/Delay  en=off  latency=1  dbl_ovrd=off  reg_retiming=off  block_type=delay
      settings: infoedit=Hardware notes: A delay line is a chain, each link of which is an SRL16 followed by a flip-flop. If register retiming is enabled, the delay line is a chain of flip-flops.  xl_area=[1 1 0 0 0 0 0]  block_version=8.2
  Inverter : xbsIndex_r4/Inverter  en=off  latency=0  dbl_ovrd=off  block_type=inv
      settings: xl_area=[0 0 0 0 0 0 0]  block_version=8.2
  Logical : xbsIndex_r4/Logical  logical_function=AND  inputs=2  en=off  latency=0  precision=Full  arith_type=Unsigned  n_bits=16  bin_pt=0  align_bp=on  dbl_ovrd=off  block_type=logical
      settings: xl_area=[1 0 0 1 0 0 0]  block_version=8.2
  Out : Outport  OutDataType=sfix(16)  OutScaling=2^0
  wires:
  Logical/1 -> Out/1
  In/1 -> Delay/1, Inverter/1
  Delay/1 -> Logical/2
  Inverter/1 -> Logical/1

== system warp_timer/Timer 0/posedge ==
  In : Inport  OutDataType=sfix(16)  OutScaling=2^0
  Delay : xbsIndex_r4/Delay  en=off  latency=1  dbl_ovrd=off  reg_retiming=off  block_type=delay
      settings: infoedit=Hardware notes: A delay line is a chain, each link of which is an SRL16 followed by a flip-flop. If register retiming is enabled, the delay line is a chain of flip-flops.  xl_area=[1 1 0 0 0 0 0]  block_version=8.2
  Inverter : xbsIndex_r4/Inverter  en=off  latency=0  dbl_ovrd=off  block_type=inv
      settings: xl_area=[0 0 0 0 0 0 0]  block_version=8.2
  Logical : xbsIndex_r4/Logical  logical_function=AND  inputs=2  en=off  latency=0  precision=Full  arith_type=Unsigned  n_bits=16  bin_pt=0  align_bp=on  dbl_ovrd=off  block_type=logical
      settings: xl_area=[1 0 0 1 0 0 0]  block_version=8.2
  Out : Outport  OutDataType=sfix(16)  OutScaling=2^0
  wires:
  Delay/1 -> Inverter/1
  Inverter/1 -> Logical/2
  In/1 -> Logical/1, Delay/1
  Logical/1 -> Out/1

== system warp_timer/Timer 0/posedge2 ==
  In : Inport  OutDataType=sfix(16)  OutScaling=2^0
  Delay : xbsIndex_r4/Delay  en=off  latency=1  dbl_ovrd=off  reg_retiming=off  block_type=delay
      settings: infoedit=Hardware notes: A delay line is a chain, each link of which is an SRL16 followed by a flip-flop. If register retiming is enabled, the delay line is a chain of flip-flops.  xl_area=[1 1 0 0 0 0 0]  block_version=8.2
  Inverter : xbsIndex_r4/Inverter  en=off  latency=0  dbl_ovrd=off  block_type=inv
      settings: xl_area=[0 0 0 0 0 0 0]  block_version=8.2
  Logical : xbsIndex_r4/Logical  logical_function=AND  inputs=2  en=off  latency=0  precision=Full  arith_type=Unsigned  n_bits=16  bin_pt=0  align_bp=on  dbl_ovrd=off  block_type=logical
      settings: xl_area=[1 0 0 1 0 0 0]  block_version=8.2
  Out : Outport  OutDataType=sfix(16)  OutScaling=2^0
  wires:
  Delay/1 -> Inverter/1
  Inverter/1 -> Logical/2
  In/1 -> Logical/1, Delay/1
  Logical/1 -> Out/1

== system warp_timer/Timer 1/S-R_Latch1 ==
  S : Inport  OutDataType=sfix(16)  OutScaling=2^0
  R : Inport  Port=2  OutDataType=sfix(16)  OutScaling=2^0
  Inverter : xbsIndex_r4/Inverter  en=off  latency=0  dbl_ovrd=off  block_type=inv
      settings: xl_area=[0 0 0 0 0 0 0]  block_version=VER_STRING_GOES_HERE
  Register : xbsIndex_r4/Register  init=0  rst=on  en=on  dbl_ovrd=off  block_type=register
      settings: xl_area=[1 1 0 0 0 0 0]  block_version=VER_STRING_GOES_HERE
  Q : Outport  OutDataType=sfix(16)  OutScaling=2^0
  wires:
  Register/1 -> Inverter/1, Q/1
  Inverter/1 -> Register/3
  S/1 -> Register/1
  R/1 -> Register/2

== system warp_timer/Timer 1/S-R_Latch2 ==
  S : Inport  OutDataType=sfix(16)  OutScaling=2^0
  R : Inport  Port=2  OutDataType=sfix(16)  OutScaling=2^0
  Inverter : xbsIndex_r4/Inverter  en=off  latency=0  dbl_ovrd=off  block_type=inv
      settings: xl_area=[0 0 0 0 0 0 0]  block_version=VER_STRING_GOES_HERE
  Register : xbsIndex_r4/Register  init=0  rst=on  en=on  dbl_ovrd=off  block_type=register
      settings: xl_area=[1 1 0 0 0 0 0]  block_version=VER_STRING_GOES_HERE
  Q : Outport  OutDataType=sfix(16)  OutScaling=2^0
  wires:
  R/1 -> Register/2
  S/1 -> Register/1
  Inverter/1 -> Register/3
  Register/1 -> Q/1, Inverter/1

== system warp_timer/Timer 1/S-R_Latch3 ==
  S : Inport  OutDataType=sfix(16)  OutScaling=2^0
  R : Inport  Port=2  OutDataType=sfix(16)  OutScaling=2^0
  Inverter : xbsIndex_r4/Inverter  en=off  latency=0  dbl_ovrd=off  block_type=inv
      settings: xl_area=[0 0 0 0 0 0 0]  block_version=VER_STRING_GOES_HERE
  Register : xbsIndex_r4/Register  init=0  rst=on  en=on  dbl_ovrd=off  block_type=register
      settings: xl_area=[1 1 0 0 0 0 0]  block_version=VER_STRING_GOES_HERE
  Q : Outport  OutDataType=sfix(16)  OutScaling=2^0
  wires:
  R/1 -> Register/2
  S/1 -> Register/1
  Inverter/1 -> Register/3
  Register/1 -> Q/1, Inverter/1

== system warp_timer/Timer 1/Sim-only Gateway In ==
  D : Inport  OutDataType=sfix(16)  OutScaling=2^0
  Disregard Subsystem : xbsIndex_r4/Disregard Subsystem  Tag=discardX  block_type=disregard
      settings: block_version=10.1.3
  Gateway In : xbsIndex_r4/Gateway In  arith_type=Boolean  n_bits=1  bin_pt=0  quantization="Round  (unbiased: +/- Inf)"  overflow=Saturate  period=1  dbl_ovrd=off  timing_constraint=None  locs_specified=off  LOCs={}  block_type=gatewayin
      settings: infoedit="Gateway in block.  Converts inputs of type Simulink integer, double and fixed point to  Xilinx fixed point type.<P><P>Hardware notes:  In hardware these blocks become top level input ports."  xl_area=[0 0 0 0 1 0 0]  block_version=10.1.3
  Q : Outport
  wires:
  Gateway In/1 -> Q/1
  D/1 -> Gateway In/1

== system warp_timer/Timer 1/Sim-only Gateway In2 ==
  D : Inport  OutDataType=sfix(16)  OutScaling=2^0
  Disregard Subsystem : xbsIndex_r4/Disregard Subsystem  Tag=discardX  block_type=disregard
      settings: block_version=10.1.3
  Gateway In : xbsIndex_r4/Gateway In  arith_type=Boolean  n_bits=1  bin_pt=0  quantization="Round  (unbiased: +/- Inf)"  overflow=Saturate  period=1  dbl_ovrd=off  timing_constraint=None  locs_specified=off  LOCs={}  block_type=gatewayin
      settings: infoedit="Gateway in block.  Converts inputs of type Simulink integer, double and fixed point to  Xilinx fixed point type.<P><P>Hardware notes:  In hardware these blocks become top level input ports."  xl_area=[0 0 0 0 1 0 0]  block_version=10.1.3
  Q : Outport
  wires:
  D/1 -> Gateway In/1
  Gateway In/1 -> Q/1

== system warp_timer/Timer 1/negedge ==
  In : Inport  OutDataType=sfix(16)  OutScaling=2^0
  Delay : xbsIndex_r4/Delay  en=off  latency=1  dbl_ovrd=off  reg_retiming=off  block_type=delay
      settings: infoedit=Hardware notes: A delay line is a chain, each link of which is an SRL16 followed by a flip-flop. If register retiming is enabled, the delay line is a chain of flip-flops.  xl_area=[1 1 0 0 0 0 0]  block_version=8.2
  Inverter : xbsIndex_r4/Inverter  en=off  latency=0  dbl_ovrd=off  block_type=inv
      settings: xl_area=[0 0 0 0 0 0 0]  block_version=8.2
  Logical : xbsIndex_r4/Logical  logical_function=AND  inputs=2  en=off  latency=0  precision=Full  arith_type=Unsigned  n_bits=16  bin_pt=0  align_bp=on  dbl_ovrd=off  block_type=logical
      settings: xl_area=[1 0 0 1 0 0 0]  block_version=8.2
  Out : Outport  OutDataType=sfix(16)  OutScaling=2^0
  wires:
  Inverter/1 -> Logical/1
  Delay/1 -> Logical/2
  In/1 -> Inverter/1, Delay/1
  Logical/1 -> Out/1

== system warp_timer/Timer 1/posedge ==
  In : Inport  OutDataType=sfix(16)  OutScaling=2^0
  Delay : xbsIndex_r4/Delay  en=off  latency=1  dbl_ovrd=off  reg_retiming=off  block_type=delay
      settings: infoedit=Hardware notes: A delay line is a chain, each link of which is an SRL16 followed by a flip-flop. If register retiming is enabled, the delay line is a chain of flip-flops.  xl_area=[1 1 0 0 0 0 0]  block_version=8.2
  Inverter : xbsIndex_r4/Inverter  en=off  latency=0  dbl_ovrd=off  block_type=inv
      settings: xl_area=[0 0 0 0 0 0 0]  block_version=8.2
  Logical : xbsIndex_r4/Logical  logical_function=AND  inputs=2  en=off  latency=0  precision=Full  arith_type=Unsigned  n_bits=16  bin_pt=0  align_bp=on  dbl_ovrd=off  block_type=logical
      settings: xl_area=[1 0 0 1 0 0 0]  block_version=8.2
  Out : Outport  OutDataType=sfix(16)  OutScaling=2^0
  wires:
  Logical/1 -> Out/1
  In/1 -> Delay/1, Logical/1
  Inverter/1 -> Logical/2
  Delay/1 -> Inverter/1

== system warp_timer/Timer 1/posedge2 ==
  In : Inport  OutDataType=sfix(16)  OutScaling=2^0
  Delay : xbsIndex_r4/Delay  en=off  latency=1  dbl_ovrd=off  reg_retiming=off  block_type=delay
      settings: infoedit=Hardware notes: A delay line is a chain, each link of which is an SRL16 followed by a flip-flop. If register retiming is enabled, the delay line is a chain of flip-flops.  xl_area=[1 1 0 0 0 0 0]  block_version=8.2
  Inverter : xbsIndex_r4/Inverter  en=off  latency=0  dbl_ovrd=off  block_type=inv
      settings: xl_area=[0 0 0 0 0 0 0]  block_version=8.2
  Logical : xbsIndex_r4/Logical  logical_function=AND  inputs=2  en=off  latency=0  precision=Full  arith_type=Unsigned  n_bits=16  bin_pt=0  align_bp=on  dbl_ovrd=off  block_type=logical
      settings: xl_area=[1 0 0 1 0 0 0]  block_version=8.2
  Out : Outport  OutDataType=sfix(16)  OutScaling=2^0
  wires:
  Logical/1 -> Out/1
  In/1 -> Delay/1, Logical/1
  Inverter/1 -> Logical/2
  Delay/1 -> Inverter/1

== system warp_timer/Timer 2/S-R_Latch1 ==
  S : Inport  OutDataType=sfix(16)  OutScaling=2^0
  R : Inport  Port=2  OutDataType=sfix(16)  OutScaling=2^0
  Inverter : xbsIndex_r4/Inverter  en=off  latency=0  dbl_ovrd=off  block_type=inv
      settings: xl_area=[0 0 0 0 0 0 0]  block_version=VER_STRING_GOES_HERE
  Register : xbsIndex_r4/Register  init=0  rst=on  en=on  dbl_ovrd=off  block_type=register
      settings: xl_area=[1 1 0 0 0 0 0]  block_version=VER_STRING_GOES_HERE
  Q : Outport  OutDataType=sfix(16)  OutScaling=2^0
  wires:
  R/1 -> Register/2
  S/1 -> Register/1
  Inverter/1 -> Register/3
  Register/1 -> Q/1, Inverter/1

== system warp_timer/Timer 2/S-R_Latch2 ==
  S : Inport  OutDataType=sfix(16)  OutScaling=2^0
  R : Inport  Port=2  OutDataType=sfix(16)  OutScaling=2^0
  Inverter : xbsIndex_r4/Inverter  en=off  latency=0  dbl_ovrd=off  block_type=inv
      settings: xl_area=[0 0 0 0 0 0 0]  block_version=VER_STRING_GOES_HERE
  Register : xbsIndex_r4/Register  init=0  rst=on  en=on  dbl_ovrd=off  block_type=register
      settings: xl_area=[1 1 0 0 0 0 0]  block_version=VER_STRING_GOES_HERE
  Q : Outport  OutDataType=sfix(16)  OutScaling=2^0
  wires:
  Register/1 -> Inverter/1, Q/1
  Inverter/1 -> Register/3
  S/1 -> Register/1
  R/1 -> Register/2

== system warp_timer/Timer 2/S-R_Latch3 ==
  S : Inport  OutDataType=sfix(16)  OutScaling=2^0
  R : Inport  Port=2  OutDataType=sfix(16)  OutScaling=2^0
  Inverter : xbsIndex_r4/Inverter  en=off  latency=0  dbl_ovrd=off  block_type=inv
      settings: xl_area=[0 0 0 0 0 0 0]  block_version=VER_STRING_GOES_HERE
  Register : xbsIndex_r4/Register  init=0  rst=on  en=on  dbl_ovrd=off  block_type=register
      settings: xl_area=[1 1 0 0 0 0 0]  block_version=VER_STRING_GOES_HERE
  Q : Outport  OutDataType=sfix(16)  OutScaling=2^0
  wires:
  Register/1 -> Inverter/1, Q/1
  Inverter/1 -> Register/3
  S/1 -> Register/1
  R/1 -> Register/2
